simulink model "DCmotor"  (R2026a)
settings: Solver=VariableStepAuto
values from neighbouring files (symbols this model uses):
  c = 8    [DCmototdata.m]    (also in dc_motor_data.m)
  I = 2    [DCmototdata.m]    (also in dc_motor_data.m)
  KT = 0.12    [DCmototdata.m]    (also in Kartdata.m; dc_motor_data.m; kartdata.m)
  KV = 0.127    [DCmototdata.m]    (also in Kartdata.m; dc_motor_data.m; kartdata.m)
  La = 0.01    [DCmototdata.m]    (also in Kartdata.m; dc_motor_data.m; kartdata.m)
  Ra = 0.053    [DCmototdata.m]    (also in Kartdata.m; dc_motor_data.m; kartdata.m)
settings Model: Creator=suria  LastModifiedBy=suria

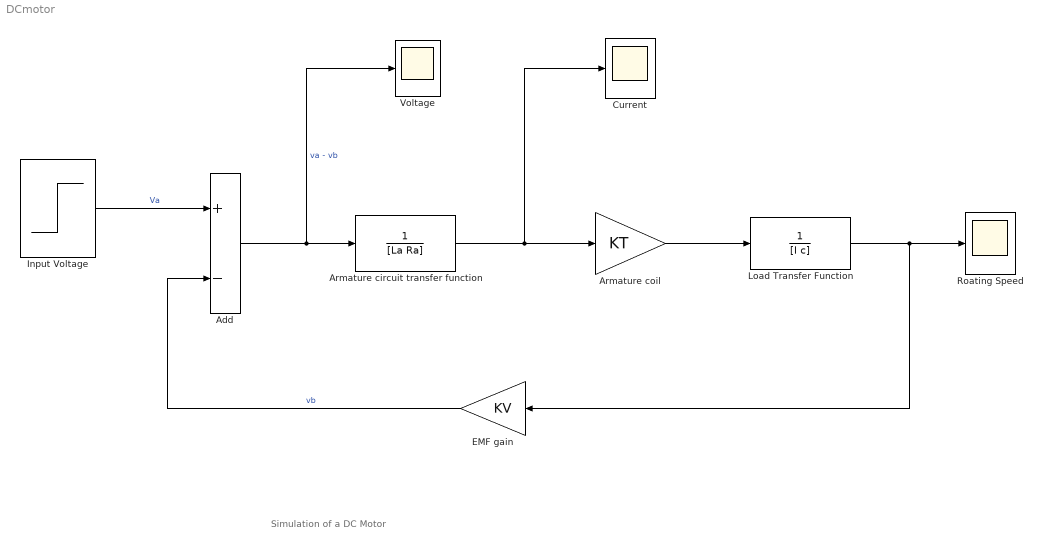
== system DCmotor ==
  note: Simulation of a DC Motor
  Add : Sum  Inputs=+-
  Armature circuit transfer function : TransferFcn  Denominator=[La Ra]
  Armature coil : Gain  Gain=KT
  Current : Scope
      settings: ActiveDisplayYMinimum=-1  ActiveDisplayYMaximum=1  DataLoggingVariableName=ScopeData2
  EMF gain : Gain  Gain=KV
  Input Voltage : Step  Time=0  FinalValue=Va  SampleTime=0
  Load Transfer Function : TransferFcn  Denominator=[I c]
  Roating Speed : Scope
      settings: ActiveDisplayYMinimum=-9.1433283291044738  ActiveDisplayYMaximum=26.638242193913371
  Voltage : Scope
      settings: ActiveDisplayYMinimum=-1  ActiveDisplayYMaximum=1
  wires:
  Input Voltage/1 -> Add/1  "Va"
  EMF gain/1 -> Add/2  "vb"
  Add/1 -> Voltage/1, Armature circuit transfer function/1  "va - vb"
  Armature circuit transfer function/1 -> Current/1, Armature coil/1
  Armature coil/1 -> Load Transfer Function/1
  Load Transfer Function/1 -> EMF gain/1, Roating Speed/1
